simulink model "P3_13"  (R2024b)
settings: Solver=VariableStepAuto  StartTime=0.0  StopTime=30  RelTol=1e-3
settings Model: Creator=Rj Avro Biswas  LastModifiedBy=Rj Avro Biswas

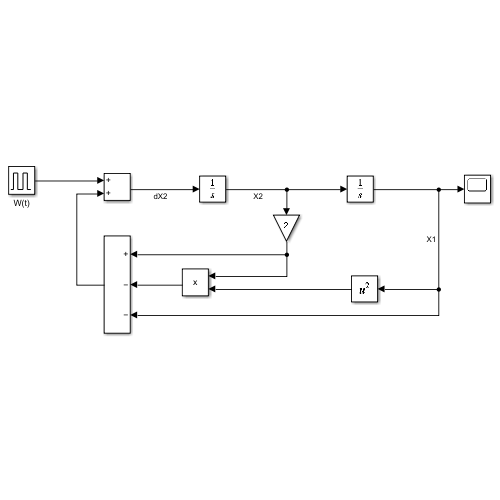
[thumbnail: Simulink's stored preview of the top-level diagram]
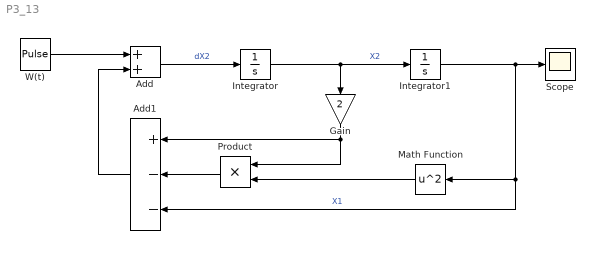
== system P3_13 ==
  Add : Sum
  Add1 : Sum  Inputs=+--
  Gain : Gain  Gain=2
  Integrator : Integrator  InitialCondition=2
  Integrator1 : Integrator  InitialCondition=-2
  Math Function : Math  Operator=square
  Product : Product
  Scope : Scope
  W(t) : DiscretePulseGenerator  PulseType=Time based  Amplitude=10  Period=10  PulseWidth=.25
  wires:
  Integrator/1 -> Integrator1/1, Gain/1  "X2"
  Add/1 -> Integrator/1  "dX2"
  W(t)/1 -> Add/1
  Add1/1 -> Add/2
  Integrator1/1 -> Add1/3, Math Function/1, Scope/1  "X1"
  Gain/1 -> Product/1, Add1/1
  Product/1 -> Add1/2
  Math Function/1 -> Product/2
